simulink model "PMSM_Motor_Model_FOC_Control"  (R2021b)
settings: Solver=VariableStepAuto  StartTime=0.0  StopTime=10.0  RelTol=1e-3
undefined symbols (not defined in the file): b, DiscIntNeverNeededParam, ee_sli_rtmsupport, fsw, gcbh, idMatrix, iqMatrix, J, Ld, Lq, ModFactor, N, PM, Pmax, psim, rpmVec, Rs, Tmax, TqVec, Ts, Tsc, VdcVec
libraries: simulink x8, eeTransforms x4, eeDiscretePi x3, autolibinverter x1
settings Model: Creator=sejal  LastModifiedBy=sejal

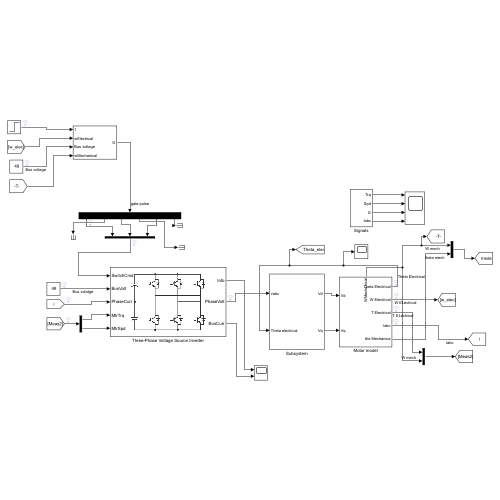
[thumbnail: Simulink's stored preview of the top-level diagram]
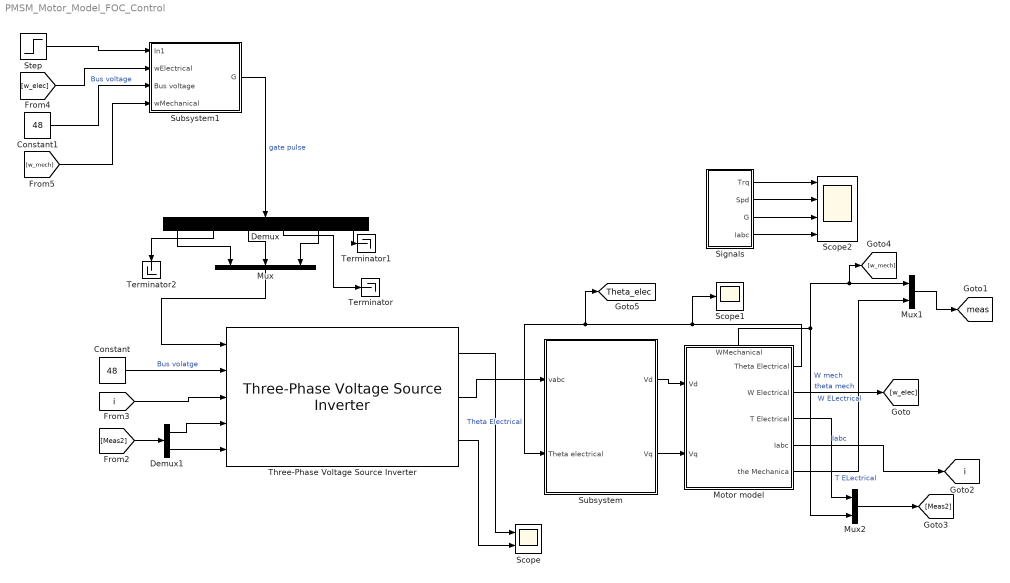
== system PMSM_Motor_Model_FOC_Control ==
  Constant : Constant  Value=48
  Constant1 : Constant  Value=48
  Demux : Demux  Outputs=6
  Demux1 : Demux  Outputs=2
  Motor model : Subsystem
      settings: PortSchema="{\"entries\":[{\"content\":{\"sides\":[{\"content\":{\"connectorIds\":[\"In1\",\"In2\"]},\"type\":\"ConnectorPlacement.EquallySpacedRectSide\",\"uuid\":\"d94b5778-ca34-457d-ba2a-6926521c1488\"},{\"content\":{\"connectorIds\":[\"Out1\",\"Out2\",\"Out3\",\"Out4\",\"Out5\"],\"side\":\"RIGHT\"},\"type\":\"ConnectorPlacement.EquallySpacedRectSide\",\"uuid\":\"5ff0fb9f-c423-410a-89d0-b078d17a40d7\"},{\"content\":{\"connectorIds\":[\"Out6\"],\"side\":\"TOP\"},\"type\":\"ConnectorPlacement.EquallySpacedRectSide\",\"uuid\":\"89b2a84c-26aa-4c46-93dc-fd6c7b13ef43\"}]},\"type\":\"ConnectorPlacement.EquallySpacedConnector\",\"uuid\":\"8745b86b-46e7-4df9-819f-71db080298ce\"}],\"packageUris\":[\"http://schema.mathworks.com/mf0/Connector/R2020b\"],\"version\":\"1.0\"}"
  Mux : Mux  Inputs=3
  Mux1 : Mux  Inputs=2
  Mux2 : Mux  Inputs=2
  Scope : Scope  NumInputPorts=2
  Scope1 : Scope
  Scope2 : Scope  NumInputPorts=4
  "Signals " : Subsystem
  Step : Step  After=500  SampleTime=0
  Subsystem : Subsystem
  Subsystem1 : Subsystem
  Terminator : Terminator
  Terminator1 : Terminator
  Terminator2 : Terminator
  Three-Phase Voltage Source Inverter : autolibinverter/Three-Phase Voltage Source Inverter  InvrtrTmpInpEnbl=off  enable_hdl=off  model_type=Switch inputs  fs=10000  w_eff_bp=[-1000 -500 0 500 1000]  n1=128  T_eff_bp=[-200 -100 0 100 200]  Temp_eff_bp=[213.15 293.15 373.15]  n2=128  ploss_table=[1 0.999 0.989 0.997 0.996;0.995 0.994 0.993 0.992 0.991;0.990 0.989 0.988 0.987 0.986;0.985 0.984 0.983 0.982 0.981;0.980 0.979 0.978 0.977 0.976]  ploss_table_3d=cat(3,0.95*[1 0.999 0.989 0.997 0.996;0.995 0.994 0.993 0.992 0.991;0.990 0.989 0.988 0.987 0.986;0.985 0.984 0.983 0.982 0.981;0.980 0.979 0.978 0.977 0.976],[1 0.999 0.989 0.997 0.996;0.995 0.994 0.993 0.992 0.991;0.990 0.989 0.988 0.987 0.986;0.985 0.984 0.983 0.982 0.981;0.980 0.979 0.978 0.977 0.976],0.92*[1 0.999 0.989 0.997 0.996;0.995 0.994 0.993 0.992 0.991;0.990 0.989 0.988 0.987 0.986;0.985 0.984 0.983 0.982 0.981;0.980 0.979 0.978 0.977 0.976])  preExtrapFlag=off  u1max=1000  u1min=-1000  u2max=200  u2min=-200  intPrec=23  RefBlkName='autolibmappedmotor/Mapped Motor'  CalLossMapData={}  CalLossWithTempMapData={}
      settings: SourceProductBaseCode=PW,DR,MT,UV,VE
  tag scope: Theta_elec=global, i=global, meas=global
  wires:
  "Signals "/2(Spd) -> Scope2/2
  "Signals "/4(Iabc) -> Scope2/4
  Motor model/6(WMechanical) -> Mux2/2, [w_mech], Mux1/1  "W mech"
  "Signals "/1(Trq) -> Scope2/1
  Three-Phase Voltage Source Inverter/2 -> Subsystem/1(vabc)
  Motor model/5(the Mechanica) -> Mux1/2  "theta mech"
  Demux/4 -> Terminator/1
  Demux/2 -> Terminator2/1
  Motor model/4(Iabc) -> [i]  "Iabc"
  Constant/1 -> Three-Phase Voltage Source Inverter/2  "Bus volatge"
  Mux2/1 -> [Meas2]
  Demux1/1 -> Three-Phase Voltage Source Inverter/4
  Demux1/2 -> Three-Phase Voltage Source Inverter/5
  [i] -> Three-Phase Voltage Source Inverter/3
  Motor model/1(Theta Electrical) -> Scope1/1, [Theta_elec], Subsystem/2(Theta electrical)  "Theta Electrical"
  Motor model/3(T Electrical) -> Mux2/1  "T ELectrical"
  Demux/1 -> Mux/1
  Demux/6 -> Terminator1/1
  Subsystem/2(Vq) -> Motor model/2(Vq)
  Three-Phase Voltage Source Inverter/3 -> Scope/2
  Three-Phase Voltage Source Inverter/1 -> Scope/1
  Subsystem/1(Vd) -> Motor model/1(Vd)
  "Signals "/3(G) -> Scope2/3
  [Meas2] -> Demux1/1
  Mux1/1 -> [meas]
  Demux/5 -> Mux/3
  Subsystem1/1(G) -> Demux/1  "gate pulse"
  Demux/3 -> Mux/2
  Mux/1 -> Three-Phase Voltage Source Inverter/1
  Motor model/2(W Electrical) -> [w_elec]  "W ELectrical"
  Step/1 -> Subsystem1/1(In1)
  [w_elec] -> Subsystem1/2(wElectrical)
  Constant1/1 -> Subsystem1/3(Bus voltage)  "Bus voltage"
  [w_mech] -> Subsystem1/4(wMechanical)

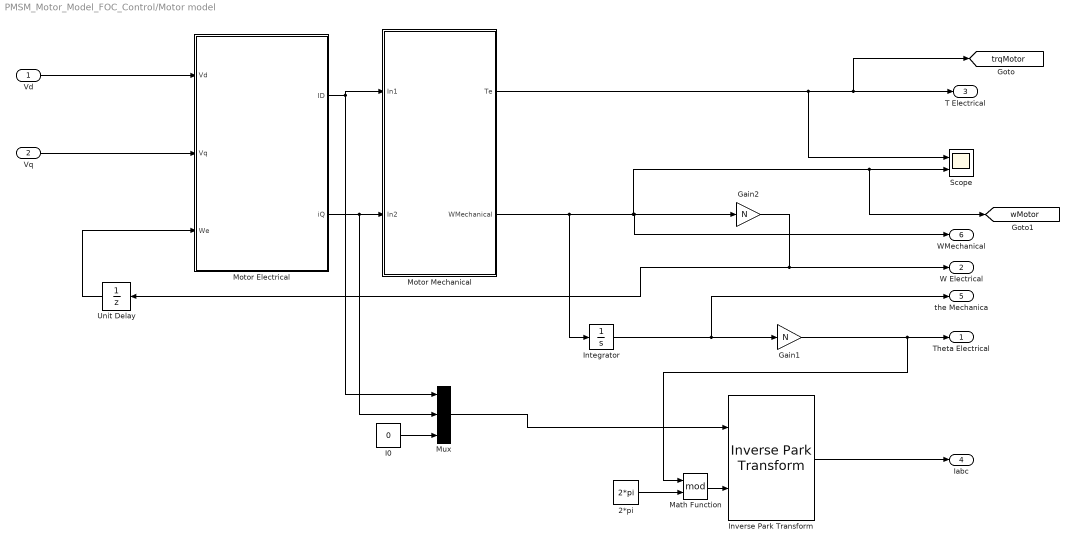
== system PMSM_Motor_Model_FOC_Control/Motor model ==
  Vd : Inport
  Vq : Inport  Port=2
  2*pi : Constant  Value=2*pi  SampleTime=Tsc
  Gain1 : Gain  Gain=N
  Gain2 : Gain  Gain=N
  I0 : Constant  Value=0
  Integrator : Integrator
  Inverse Park Transform : eeTransforms/Inverse Park Transform  AxisAlignment=Q-axis  PowerInvariant=off
  Math Function : Math  Operator=mod  SignedPower=on  SaturateOnIntegerOverflow=on
  Motor Electrical : Subsystem
  Motor Mechanical : Subsystem
  Mux : Mux  Inputs=3
  Scope : Scope  NumInputPorts=2
  Unit Delay : UnitDelay  SampleTime=-1  HasFrameUpgradeWarning=on
  Theta Electrical : Outport
  W Electrical : Outport  Port=2
  T Electrical : Outport  Port=3
  Iabc : Outport  Port=4
  the Mechanica : Outport  Port=5
  WMechanical : Outport  Port=6
  tag scope: trqMotor=global, wMotor=global
  wires:
  Motor Electrical/2(iQ) -> Mux/2, Motor Mechanical/2(In2)
  Motor Electrical/1(ID) -> Motor Mechanical/1(In1), Mux/1
  Vd/1 -> Motor Electrical/1(Vd)
  Motor Mechanical/1(Te) -> Scope/1, [trqMotor], T Electrical/1
  Vq/1 -> Motor Electrical/2(Vq)
  Integrator/1 -> the Mechanica/1, Gain1/1
  Motor Mechanical/2(WMechanical) -> WMechanical/1, Gain2/1, [wMotor], Scope/2, Integrator/1
  Mux/1 -> Inverse Park Transform/1
  I0/1 -> Mux/3
  Inverse Park Transform/1 -> Iabc/1
  Gain2/1 -> Unit Delay/1, W Electrical/1
  Unit Delay/1 -> Motor Electrical/3(We)
  2*pi/1 -> Math Function/2
  Gain1/1 -> Math Function/1, Theta Electrical/1
  Math Function/1 -> Inverse Park Transform/2

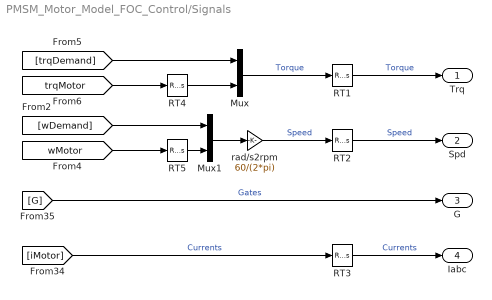
== system PMSM_Motor_Model_FOC_Control/Signals  ==
  Mux : Mux  Inputs=2
  Mux1 : Mux  Inputs=2
  RT1 : RateTransition  OutPortSampleTime=Ts
  RT2 : RateTransition  OutPortSampleTime=Ts
  RT3 : RateTransition  OutPortSampleTime=Ts
  RT4 : RateTransition  OutPortSampleTime=Tsc
  RT5 : RateTransition  OutPortSampleTime=Tsc
  rad/s2rpm : Gain  Gain=60/(2*pi)
  Trq : Outport  VectorParamsAs1DForOutWhenUnconnected=off
  Spd : Outport  Port=2  VectorParamsAs1DForOutWhenUnconnected=off
  G : Outport  Port=3  VectorParamsAs1DForOutWhenUnconnected=off
  Iabc : Outport  Port=4  VectorParamsAs1DForOutWhenUnconnected=off
  wires:
  [trqDemand] -> Mux/1
  [G] -> G/1  "Gates"
  Mux1/1 -> rad/s2rpm/1
  Mux/1 -> RT1/1  "Torque"
  [iMotor] -> RT3/1  "Currents"
  [wDemand] -> Mux1/1
  rad/s2rpm/1 -> RT2/1  "Speed"
  [trqMotor] -> RT4/1
  [wMotor] -> RT5/1
  RT1/1 -> Trq/1  "Torque"
  RT2/1 -> Spd/1  "Speed"
  RT3/1 -> Iabc/1  "Currents"
  RT4/1 -> Mux/2
  RT5/1 -> Mux1/2

== system PMSM_Motor_Model_FOC_Control/Subsystem ==
  vabc : Inport
  Theta electrical : Inport  Port=2
  2*pi : Constant  Value=2*pi  SampleTime=Tsc
  Demux1 : Demux  Outputs=3
  Math Function : Math  Operator=mod  SignedPower=on  SaturateOnIntegerOverflow=on
  Park Transform2 : eeTransforms/Park Transform  AxisAlignment=Q-axis  PowerInvariant=off
  Terminator1 : Terminator
  Trigonometric Function : Trigonometry  Commented=on
  Trigonometric Function1 : Trigonometry  Commented=on  Operator=cos
  Vd : Outport
  Vq : Outport  Port=2
  wires:
  vabc/1 -> Park Transform2/1
  Park Transform2/1 -> Demux1/1
  Demux1/3 -> Terminator1/1
  Demux1/2 -> Vq/1
  Demux1/1 -> Vd/1
  2*pi/1 -> Math Function/2
  Theta electrical/1 -> Math Function/1
  Math Function/1 -> Park Transform2/2

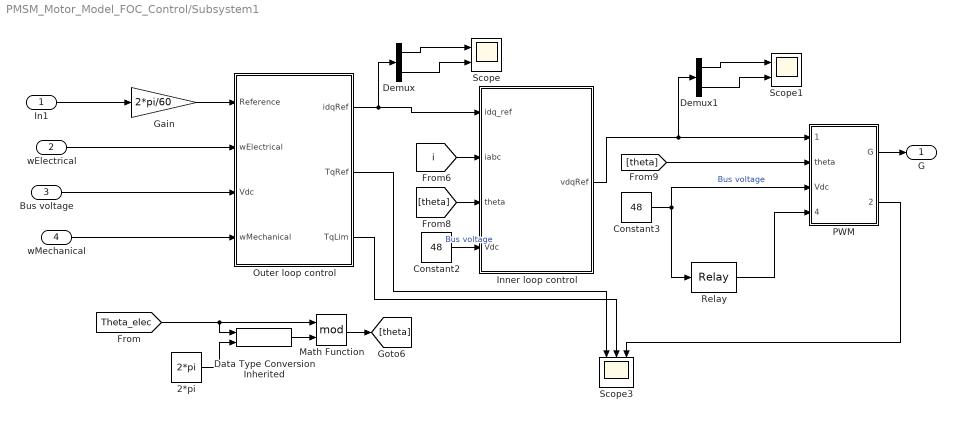
== system PMSM_Motor_Model_FOC_Control/Subsystem1 ==
  In1 : Inport
  wElectrical : Inport  Port=2
  Bus voltage : Inport  Port=3
  wMechanical : Inport  Port=4
  2*pi : Constant  Value=2*pi  OutDataTypeStr=Inherit: Inherit via back propagation  SampleTime=Tsc
  Constant2 : Constant  Value=48
  Constant3 : Constant  Value=48
  Data Type Conversion Inherited : simulink/Signal Attributes/Data Type Conversion Inherited  ConvertRealWorld=Real World Value  DoSatur=off
      settings: SourceProductBaseCode=SL
  Demux : Demux  Outputs=2
  Demux1 : Demux  Outputs=2
  Gain : Gain  Gain=2*pi/60
  Inner loop control : Subsystem  AncestorBlock=Inner_loop/Inner loop control
  Math Function : Math  Operator=mod  SignedPower=on  SaturateOnIntegerOverflow=on
  Outer loop control : Subsystem  AncestorBlock=Outer_loop/Outer loop control
  PWM : Subsystem  AncestorBlock=eePmsmFieldOrientedControl/PMSM Field-Oriented Control/PWM
  Relay : Relay  OnSwitchValue=48  OffSwitchValue=0.5*48
  Scope : Scope  NumInputPorts=2
  Scope1 : Scope  NumInputPorts=2
  Scope3 : Scope  NumInputPorts=3
  G : Outport
  wires:
  wElectrical/1 -> Outer loop control/2(wElectrical)
  [theta] -> Inner loop control/3(theta)
  Outer loop control/3(TqLim) -> Scope3/2
  Relay/1 -> PWM/4(PwmEnable)
  Data Type Conversion Inherited/1 -> Math Function/2
  In1/1 -> Gain/1
  PWM/2(ModWave) -> Scope3/3
  Gain/1 -> Outer loop control/1(Reference)
  [Theta_elec] -> Math Function/1, Data Type Conversion Inherited/1
  Outer loop control/1(idqRef) -> Demux/1, Inner loop control/1(idq_ref)
  Constant3/1 -> PWM/3(Vdc), Relay/1  "Bus voltage"
  [theta] -> PWM/2(theta)
  PWM/1(G) -> G/1
  [i] -> Inner loop control/2(iabc)
  Constant2/1 -> Inner loop control/4(Vdc)  "Bus voltage"
  2*pi/1 -> Data Type Conversion Inherited/2
  Outer loop control/2(TqRef) -> Scope3/1
  Math Function/1 -> [theta]
  wMechanical/1 -> Outer loop control/4(wMechanical)
  Bus voltage/1 -> Outer loop control/3(Vdc)
  Demux/1 -> Scope/1
  Demux/2 -> Scope/2
  Demux1/1 -> Scope1/1
  Inner loop control/1(vdqRef) -> Demux1/1, PWM/1(vdqRef)
  Demux1/2 -> Scope1/2

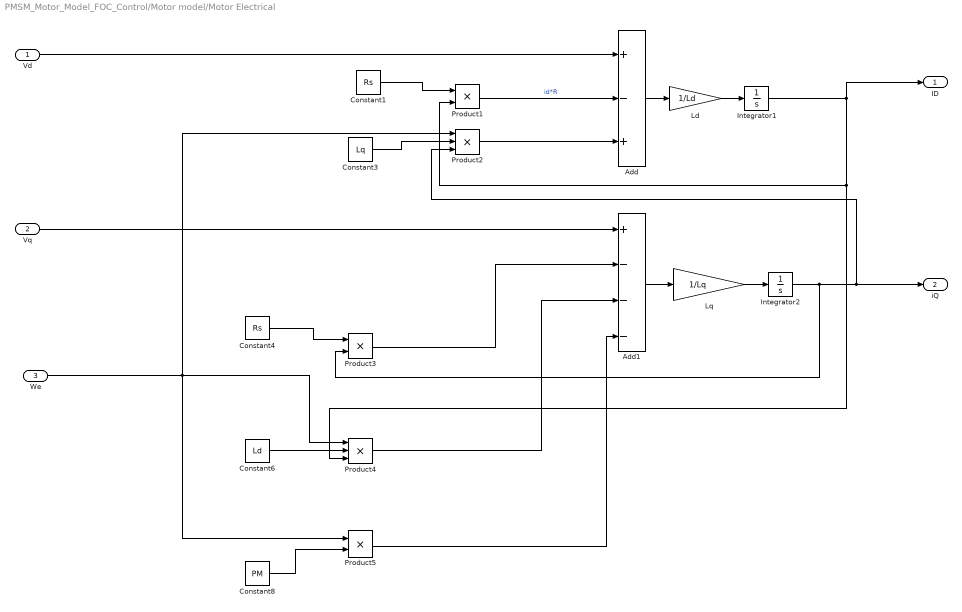
== system PMSM_Motor_Model_FOC_Control/Motor model/Motor Electrical ==
  Vd : Inport
  Vq : Inport  Port=2
  We : Inport  Port=3
  Add : Sum  Inputs=+-+
  Add1 : Sum  Inputs=+---
  Constant1 : Constant  Value=Rs
  Constant3 : Constant  Value=Lq
  Constant4 : Constant  Value=Rs
  Constant6 : Constant  Value=Ld
  Constant8 : Constant  Value=PM
  Integrator1 : Integrator
  Integrator2 : Integrator
  Ld : Gain  Gain=1/Ld
  Lq : Gain  Gain=1/Lq
  Product1 : Product
  Product2 : Product  Inputs=3
  Product3 : Product
  Product4 : Product  Inputs=3
  Product5 : Product
  ID : Outport
  iQ : Outport  Port=2
  wires:
  Constant3/1 -> Product2/2
  Add/1 -> Ld/1
  Product5/1 -> Add1/4
  Integrator2/1 -> Product2/3, iQ/1, Product3/2
  Constant8/1 -> Product5/2
  Constant1/1 -> Product1/1
  Product1/1 -> Add/2  "id*R"
  Product2/1 -> Add/3
  Add1/1 -> Lq/1
  We/1 -> Product5/1, Product2/1, Product4/1
  Constant4/1 -> Product3/1
  Lq/1 -> Integrator2/1
  Product3/1 -> Add1/2
  Constant6/1 -> Product4/2
  Product4/1 -> Add1/3
  Vd/1 -> Add/1
  Vq/1 -> Add1/1
  Integrator1/1 -> Product1/2, Product4/3, ID/1
  Ld/1 -> Integrator1/1

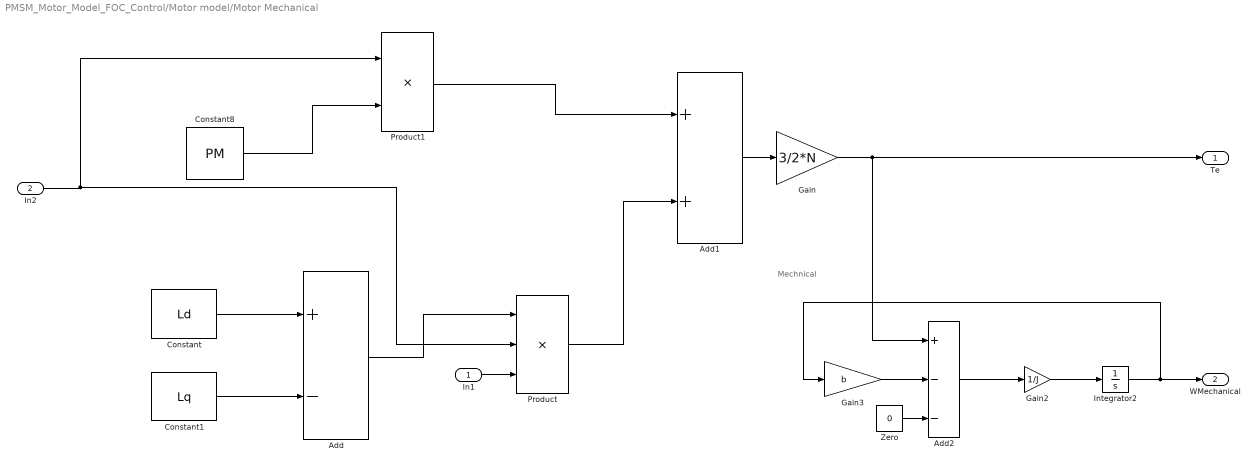
== system PMSM_Motor_Model_FOC_Control/Motor model/Motor Mechanical ==
  note: Mechnical
  In1 : Inport
  In2 : Inport  Port=2
  Add : Sum  Inputs=+-
  Add1 : Sum
  Add2 : Sum  Inputs=+--
  Constant : Constant  Value=Ld
  Constant1 : Constant  Value=Lq
  Constant8 : Constant  Value=PM
  Gain : Gain  Gain=3/2*N
  Gain2 : Gain  Gain=1/J
  Gain3 : Gain  Gain=b
  Integrator2 : Integrator
  Product : Product  Inputs=3
  Product1 : Product
  Zero : Constant  Value=0  OutDataTypeStr=Inherit: Inherit via back propagation
  Te : Outport
  WMechanical : Outport  Port=2
  wires:
  Add1/1 -> Gain/1
  Constant8/1 -> Product1/2
  Constant/1 -> Add/1
  Add/1 -> Product/1
  Constant1/1 -> Add/2
  Product1/1 -> Add1/1
  Product/1 -> Add1/2
  In2/1 -> Product/2, Product1/1
  In1/1 -> Product/3
  Gain/1 -> Te/1, Add2/1
  Zero/1 -> Add2/3
  Gain3/1 -> Add2/2
  Integrator2/1 -> WMechanical/1, Gain3/1
  Add2/1 -> Gain2/1
  Gain2/1 -> Integrator2/1

== system PMSM_Motor_Model_FOC_Control/Subsystem1/Inner loop control ==
  idq_ref : Inport
  iabc : Inport  Port=2
  theta : Inport  Port=3
  Vdc : Inport  Port=4
  Constant : Constant  Value=0  SampleTime=-1
  Gain : Gain  Gain=1/sqrt(3)
  PMSM Current Controller : Subsystem  AncestorBlock=eePmsmCurrentController/PMSM Current Controller  LoadFcn=ee_sli_rtmsupport( 'loadfcn', gcbh );  mask(PMSM Current Controller){Kp_id=0.1, Ki_id=10, Kaw_id=1000, Kp_iq=0.1, Ki_iq=10, Kaw_iq=1000, Ts=-1, Tsd=0.001, AxisPrio=Q-axis, ActZC=off, ActFF=on}
      mask prompts: Kp_id "physmod:ee:library:comments:control:eePmsmCurrentController:DaxisCurrentProportionalGain_MP"; Ki_id "physmod:ee:library:comments:control:eePmsmCurrentController:DaxisCurrentIntegralGain_MP"; Kaw_id "physmod:ee:library:comments:control:eePmsmCurrentController:DaxisCurrentAntiwindupGain_MP"; Kp_iq "physmod:ee:library:comments:control:eePmsmCurrentController:QaxisCurrentProportionalGain_MP"; Ki_iq "physmod:ee:library:comments:control:eePmsmCurrentController:QaxisCurrentIntegralGain_MP"; Kaw_iq "physmod:ee:library:comments:control:eePmsmCurrentController:QaxisCurrentAntiwindupGain_MP"; Ts "physmod:ee:library:comments:control:eePmsmCurrentController:SampleTime1ForInherited_MP"; Tsd "physmod:ee:library:comments:control:eePmsmCurrentController:DiscretizationSampleTime_MP"; AxisPrio "physmod:ee:library:comments:control:eePmsmCurrentController:AxisPrioritization_MP"; ActZC "physmod:ee:library:comments:control:eePmsmCurrentController:EnableZeroCancellation_MP"; ActFF "physmod:ee:library:comments:control:eePmsmCurrentController:EnablePrecontrolVoltage_MP"
      mask help: physmod:ee:library:comments:control:eePmsmCurrentController:PMSMCurrentController_MD
      mask init:
      | [Tsd, numZC_id, denZC_id, numZC_iq, denZC_iq] = ee.mask.initializePmsmCurrentController(ActZC,Ts,Tsd,Kp_id,Ki_id,Kp_iq,Ki_iq);
      settings: CopyFcn=ee_sli_rtmsupport( 'copyfcn', gcbh );  DeleteFcn=ee_sli_rtmsupport( 'deletefcn', gcbh );  ModelCloseFcn=ee_sli_rtmsupport( 'modelclosefcn', gcbh );  PostSaveFcn=ee_sli_rtmsupport( 'postsavefcn', gcbh );  PreCopyFcn=ee_sli_rtmsupport( 'precopyfcn', gcbh );  OpenFcn=ee_sli_rtmsupport( 'openfcn', gcbh );  CloseFcn=ee_sli_rtmsupport( 'closefcn', gcbh );  PreDeleteFcn=ee_sli_rtmsupport( 'predeletefcn', gcbh );
      mask Help: web(nesl_help(gcbh))
      mask Callback Ts: ee.mask.callbackZeroCancellation(gcb);
      mask TypeOptions AxisPrio: d-q Voltage Limiter/AxisPrio
      mask Callback ActZC: ee.mask.callbackZeroCancellation(gcb);
      mask DialogControl Container1 Prompt: physmod:ee:library:comments:control:eePmsmCurrentController:tab_ControlParameters
      mask DialogControl Kp_id Prompt: D-axis current proportional gain
      mask DialogControl Ki_id Prompt: D-axis current integral gain
      mask DialogControl Kaw_id Prompt: D-axis current anti-windup gain
      mask DialogControl Kp_iq Prompt: Q-axis current proportional gain
      mask DialogControl Ki_iq Prompt: Q-axis current integral gain
      mask DialogControl Kaw_iq Prompt: Q-axis current anti-windup gain
      mask DialogControl Ts Prompt: Sample time (-1 for inherited)
      mask DialogControl Tsd Prompt: Discretization sample time
      mask DialogControl AxisPrio Prompt: Axis prioritization
      mask DialogControl ActZC Prompt: Enable zero cancellation
      mask DialogControl ActFF Prompt: Enable pre-control voltage
  Park Transform : eeTransforms/Park Transform  AxisAlignment=Q-axis  PowerInvariant=off
  vdqRef : Outport  VectorParamsAs1DForOutWhenUnconnected=off
  wires:
  idq_ref/1 -> PMSM Current Controller/1(idqRef)
  iabc/1 -> Park Transform/1
  Vdc/1 -> Gain/1
  PMSM Current Controller/1(vdqRef) -> vdqRef/1
  theta/1 -> Park Transform/2
  Park Transform/1 -> PMSM Current Controller/2(idq)
  Constant/1 -> PMSM Current Controller/4(Reset)
  Gain/1 -> PMSM Current Controller/3(VphMax)

== system PMSM_Motor_Model_FOC_Control/Subsystem1/Outer loop control ==
  Reference : Inport
  wElectrical : Inport  Port=2
  Vdc : Inport  Port=3
  wMechanical : Inport  Port=4  SampleTime=Ts
  Discrete PI Controller : eeDiscretePi/Discrete PI Controller  Kp=60  Ki=300*2  Kaw=1000  x0=0  Ts=Ts
      settings: SourceProductBaseCode=PS
  PMSM Current Reference Generator : Subsystem  AncestorBlock=eePmsmCurrentReferenceGen/PMSM Current Reference Generator  LoadFcn=ee_sli_rtmsupport( 'loadfcn', gcbh );  mask(PMSM Current Reference Generator){Vnom=48, Pmax=Pmax, Tmax=Tmax, Ts=Tsc, RefType=Zero d-axis control, rpmVec=rpmVec, TqVec=TqVec, VdcVec=VdcVec, PWMMode=SVM: space vector modulation, ModFactor=ModFactor, idMatrix=idMatrix, iqMatrix=iqMatrix, p=N, psim=psim, Ld=Ld, Lq=Lq, Rs=Rs, RefExpEnable=0}
      mask prompts: Vnom "physmod:ee:library:comments:control:eePmsmCurrentReferenceGen:NominalDclinkVoltageV_MP"; Pmax "physmod:ee:library:comments:control:eePmsmCurrentReferenceGen:MaximumPowerW_MP"; Tmax "physmod:ee:library:comments:control:eePmsmCurrentReferenceGen:MaximumTorqueNm_MP"; Ts "physmod:ee:library:comments:control:eePmsmCurrentReferenceGen:SampleTime1ForInherited_MP"; RefType "physmod:ee:library:comments:control:eePmsmCurrentReferenceGen:CurrentReferences_MP"; rpmVec "physmod:ee:library:comments:control:eePmsmCurrentReferenceGen:MechanicalSpeedVectorWMechanicalrpm_MP"; TqVec "physmod:ee:library:comments:control:eePmsmCurrentReferenceGen:TorqueReferenceVectorTqRefNm_MP"; VdcVec "physmod:ee:library:comments:control:eePmsmCurrentReferenceGen:DClinkVoltageVectorVdcV_MP"; PWMMode "physmod:ee:library:comments:control:eePmsmCurrentReferenceGen:PWMMethod_MP"; ModFactor "physmod:ee:library:comments:control:eePmsmCurrentReferenceGen:ModulationFactor_MP"; idMatrix "physmod:ee:library:comments:control:eePmsmCurrentReferenceGen:DaxisCurrentReferenceMatrixIdwMechanicalTqRefVdcA_MP"; iqMatrix "physmod:ee:library:comments:control:eePmsmCurrentReferenceGen:QaxisCurrentReferenceMatrixIqwMechanicalTqRefVdcA_MP"; p "physmod:ee:library:comments:control:eePmsmCurrentReferenceGen:NumberOfRotorPolePairs_MP"; psim "physmod:ee:library:comments:control:eePmsmCurrentReferenceGen:PermanentMagnetFluxLinkageWb_MP"; Ld "physmod:ee:library:comments:control:eePmsmCurrentReferenceGen:DaxisInductanceH_MP"; Lq "physmod:ee:library:comments:control:eePmsmCurrentReferenceGen:QaxisInductanceH_MP"; Rs "physmod:ee:library:comments:control:eePmsmCurrentReferenceGen:StatorResistanceOhm_MP"; RefExpEnable "physmod:ee:library:comments:control:eePmsmCurrentReferenceGen:ExportCurrentReferences_MP"
      mask help: physmod:ee:library:comments:control:eePmsmCurrentReferenceGen:PMSMCurrentReferenceGenerator_MD
      mask init:
      | if Vnom <= 0            
      |     error(message('physmod:simscape:compiler:patterns:checks:GreaterThanZero',getString(message('physmod:ee:library:comments:control:eePmsmCurrentReferenceGen:NominalDclinkVoltageV_MP'))));            
      | end
      | if Pmax <= 0            
      |     error(message('physmod:simscape:compiler:patterns:checks:GreaterThanZero',getString(message('physmod:ee:library:comments:control:eePmsmCurrentReferenceGen:MaximumPowerW_MP'))));            
      | end
      | if Tmax <= 0            
      |     error(message('physmod:simscape:compiler:patterns:checks:GreaterThanZero',getString(message('physmod:ee:library:comments:control:eePmsmCurrentReferenceGen:MaximumTorqueNm_MP'))));            
      | end
      | switch RefType
      |     case 'Zero d-axis control'
      |         EnableZDAC = 1;
      |         rpmVec = [0, 3000];
      |         TqVec  = [-100, 0, 100];
      |         VdcVec = [300, 350];
      |         idMatrix = zeros(2,3,2);
      |         iqMatrix = zeros(2,3,2);
      |     case 'Lookup-table based'
      |         EnableZDAC = 0;
      |         if length(rpmVec) < 2            
      |             error(message('physmod:simscape:compiler:patterns:checks:LengthGreaterThanOrEqual',getString(message('physmod:ee:library:comments:control:eePmsmCurrentReferenceGen:MechanicalSpeedVectorWMechanicalrpm_MP')), '2'));            
      |         end
      |         if ~all(diff(rpmVec) > 0)            
      |             error(message('physmod:simscape:compiler:patterns:checks:StrictlyAscendingVec',getString(message('physmod:ee:library:comments:control:eePmsmCurrentReferenceGen:MechanicalSpeedVectorWMechanicalrpm_MP'))));            
      |         end
      |         if length(TqVec) < 2            
      |             error(message('physmod:simscape:compiler:patterns:checks:LengthGreaterThanOrEqual',getString(message('physmod:ee:library:comments:control:eePmsmCurrentReferenceGen:TorqueReferenceVectorTqRefNm_MP')), '2'));            
      |         end
      |         if ~all(diff(TqVec) > 0)            
      |             error(message('physmod:simscape:compiler:patterns:checks:StrictlyAscendingVec',getString(message('physmod:ee:library:comments:control:eePmsmCurrentReferenceGen:TorqueReferenceVectorTqRefNm_MP'))));            
      |         end
      |         if length(VdcVec) < 2            
      |             error(message('physmod:simscape:compiler:patterns:checks:LengthGreaterThanOrEqual',getString(message('physmod:ee:library:comments:control:eePmsmCurrentReferenceGen:DClinkVoltageVectorVdcV_MP')), '2'));            
      |         end
      |         if ~all(diff(VdcVec) > 0)            
      |             error(message('physmod:simscape:compiler:patterns:checks:StrictlyAscendingVec',getString(message('physmod:ee:library:comments:control:eePmsmCurrentReferenceGen:DClinkVoltageVectorVdcV_MP'))));            
      |         end
      |         if ~all(size(idMatrix) == [length(rpmVec), length(TqVec), length(VdcVec)])            
      |             error(message('physmod:simscape:compiler:patterns:checks:Size3DEqual',getString(message('physmod:ee:library:comments:control:eePmsmCurrentReferenceGen:DaxisCurrentReferenceMatrixIdwMechanicalTqRefVdcA_MP')), getString(message('physmod:ee:library:comments:control:eePmsmCurrentReferenceGen:MechanicalSpeedVectorWMechanicalrpm_MP')), getString(message('physmod:ee:library:comments:control:eePmsmCurrentReferenceGen:TorqueReferenceVectorTqRefNm_MP')), getString(message('physmod:ee:library:comments:control:eePmsmCurrentReferenceGen:DClinkVoltageVectorVdcV_MP'))));            
      |         end
      |         if ~all(size(iqMatrix) == [length(rpmVec), length(TqVec), length(VdcVec)])            
      |             error(message('physmod:simscape:compiler:patterns:checks:Size3DEqual',getString(message('physmod:ee:library:comments:control:eePmsmCurrentReferenceGen:QaxisCurrentReferenceMatrixIqwMechanicalTqRefVdcA_MP')), getString(message('physmod:ee:library:comments:control:eePmsmCurrentReferenceGen:MechanicalSpeedVectorWMechanicalrpm_MP')), getString(message('physmod:ee:library:comments:control:eePmsmCurrentReferenceGen:TorqueReferenceVectorTqRefNm_MP')), getString(message('physmod:ee:library:comments:control:eePmsmCurrentReferenceGen:DClinkVoltageVectorVdcV_MP'))));            
      |         end
      |     case 'Automatically generated lookup-table'
      |         EnableZDAC = 0;
      |         if Rs <= 0            
      |             error(message('physmod:simscape:compiler:patterns:checks:GreaterThanZero',getString(message('physmod:ee:library:comments:control:eePmsmCurrentReferenceGen:StatorResistanceOhm_MP'))));            
      |         end
      |         if Ld <= 0            
      |             error(message('physmod:simscape:compiler:patterns:checks:GreaterThanZero',getString(message('physmod:ee:library:comments:control:eePmsmCurrentReferenceGen:DaxisInductanceH_MP'))));            
      |         end
      |         if Lq <= 0            
      |             error(message('physmod:simscape:compiler:patterns:checks:GreaterThanZero',getString(message('physmod:ee:library:comments:control:eePmsmCurrentReferenceGen:QaxisInductanceH_MP'))));            
      |         end
      |         
      |         if ModFactor <= 0            
      |             error(message('physmod:simscape:compiler:patterns:checks:GreaterThanZero',getString(message('physmod:ee:library:comments:control:eePmsmCurrentReferenceGen:ModulationFactor_MP'))));            
      |         end
      |         
      |         if ModFactor > 1            
      |             error(message('physmod:simscape:compiler:patterns:checks:LessThanOrEqual',getString(message('physmod:ee:library:comments:control:eePmsmCurrentReferenceGen:ModulationFactor_MP')),'1'));            
      |         end
      |         
      |         % Check if machine parameters were changed
      |         if exist('pmsm_data', 'var')
      |             dataUpdate = (pmsm_data.Ld   ~= Ld)   ||...
      |                          (pmsm_data.Lq   ~= Lq)   ||...
      |                          (pmsm_data.psim ~= psim) ||...
      |                          (pmsm_data.p    ~= p)    ||...
      |                          (pmsm_data.Rs   ~= Rs)   ||...
      |                          (pmsm_data.Pmax ~= Pmax) ||...
      |                          (pmsm_data.Tmax ~= Tmax) ||...
      |                          (pmsm_data.PWMMode ~= PWMMode) ||...
      |                          (pmsm_data.ModFactor ~= ModFactor);
      |         end
      |         % Check if grid points were changed
      |         if exist('grid_points', 'var')
      |             VecUpdate = max(abs(grid_points.RPM_VECT - rpmVec))~=0 ||...
      |                         max(abs(grid_points.TQ_VECT  - TqVec)) ~=0 ||...
      |                         max(abs(grid_points.VDC_VECT - VdcVec))~=0;
      |         end
      |         % Compute current references only IF current references do not exist OR 
      |         % machine parameters were changed OR grid points were changed
      |         if ~exist('pmsm_ref', 'var') || dataUpdate || VecUpdate
      |             grid_points.RPM_VECT = rpmVec;
      |             grid_points.TQ_VECT  = TqVec;
      |             grid_points.VDC_VECT = VdcVec;
      |             pmsm_data.Ld    = Ld; 
      |             pmsm_data.Lq    = Lq; 
      |             pmsm_data.psim  = psim;   
      |             pmsm_data.p     = p;         
      |             pmsm_data.Rs    = Rs;   
      |             pmsm_data.Pmax  = Pmax;      
      |             pmsm_data.Tbase = Tmax;    
      |             pmsm_data.PWMMode   = PWMMode;      
      |             pmsm_data.ModFactor = ModFactor;
      |             pmsm_ref = ee.control.pmsm.getCurrentReferencesPmsm ( pmsm_data, grid_points );
      |             idMatrix = pmsm_ref.idMatrix;
      |             iqMatrix = pmsm_ref.iqMatrix;
      |         end
      |         % Export current references to base workspace
      |         if RefExpEnable==1
      |             assignin('base', 'pmsm_ref', pmsm_ref)
      |             set_param(gcb,'RefExpEnable','0');
      |         end
      | end
      settings: CopyFcn=ee_sli_rtmsupport( 'copyfcn', gcbh );  DeleteFcn=ee_sli_rtmsupport( 'deletefcn', gcbh );  ModelCloseFcn=ee_sli_rtmsupport( 'modelclosefcn', gcbh );  PostSaveFcn=ee_sli_rtmsupport( 'postsavefcn', gcbh );  PreCopyFcn=ee_sli_rtmsupport( 'precopyfcn', gcbh );  OpenFcn=ee_sli_rtmsupport( 'openfcn', gcbh );  CloseFcn=ee_sli_rtmsupport( 'closefcn', gcbh );  PreDeleteFcn=ee_sli_rtmsupport( 'predeletefcn', gcbh );
      mask Help: web(nesl_help(gcbh))
      mask TypeOptions RefType: physmod:ee:library:comments:control:eePmsmCurrentReferenceGen:ZeroD0x2DAxisControl_PV | physmod:ee:library:comments:control:eePmsmCurrentReferenceGen:Lookup0x2DTableBased_PV | physmod:ee:library:comments:control:eePmsmCurrentReferenceGen:AutomaticallyGeneratedLookup0x2DTable_PV
      mask Callback RefType:
      | % Callback function to set the parameters visibility
      | ee.mask.callbackPopupRefGenPmsm(gcb);
      mask TypeOptions PWMMode: physmod:ee:library:comments:control:eePmsmCurrentReferenceGen:SPWMSinusoidalPWM_PV | physmod:ee:library:comments:control:eePmsmCurrentReferenceGen:SVMSpaceVectorModulation_PV
      mask DialogControl Container2 Prompt: physmod:ee:library:comments:control:eePmsmCurrentReferenceGen:tab_GeneralParameters
      mask DialogControl Vnom Prompt: Nominal dc-link voltage (V)
      mask DialogControl Pmax Prompt: Maximum power (W)
      mask DialogControl Tmax Prompt: Maximum torque (N*m)
      mask DialogControl Ts Prompt: Sample time (-1 for inherited)
      mask DialogControl Container3 Prompt: physmod:ee:library:comments:control:eePmsmCurrentReferenceGen:tab_ReferenceGenStrategy
      mask DialogControl RefType Prompt: Current references
      mask DialogControl rpmVec Prompt: Mechanical speed vector, wMechanical (rpm)
      mask DialogControl TqVec Prompt: Torque reference vector, TqRef (N*m)
      mask DialogControl VdcVec Prompt: DC-link voltage vector, Vdc (V)
      mask DialogControl PWMMode Prompt: PWM method
      mask DialogControl ModFactor Prompt: Modulation factor
      mask DialogControl idMatrix Prompt: D-axis current reference matrix, id(wMechanical,TqRef,Vdc), (A)
      mask DialogControl iqMatrix Prompt: Q-axis current reference matrix, iq(wMechanical,TqRef,Vdc), (A)
      mask DialogControl p Prompt: Number of rotor pole pairs
      mask DialogControl psim Prompt: Permanent magnet flux linkage (Wb)
      mask DialogControl Ld Prompt: D-axis inductance (H)
      mask DialogControl Lq Prompt: Q-axis inductance (H)
      mask DialogControl Rs Prompt: Stator resistance (Ohm)
      mask DialogControl RefExp Prompt: physmod:ee:library:comments:control:eePmsmCurrentReferenceGen:ExportCurrentReferencesToWorkspace_B
      mask DialogControl RefExp Callback:
      | % Enable export of current references
      | set_param(gcb,'RefExpEnable','1');
      mask DialogControl RefExpEnable Prompt: Export current references
  Sum : Sum  Inputs=|+-
  Zero : Constant  Value=0  OutDataTypeStr=Inherit: Inherit via back propagation
  elec->mech : Gain  Gain=1/N
  idqRef : Outport  VectorParamsAs1DForOutWhenUnconnected=off
  TqRef : Outport  Port=2  VectorParamsAs1DForOutWhenUnconnected=off
  TqLim : Outport  Port=3  VectorParamsAs1DForOutWhenUnconnected=off
  wires:
  wMechanical/1 -> Sum/2
  Sum/1 -> Discrete PI Controller/1
  Zero/1 -> Discrete PI Controller/3, Discrete PI Controller/2
  Discrete PI Controller/1 -> PMSM Current Reference Generator/1(TqRef)  "Torque reference"
  Reference/1 -> Sum/1
  wElectrical/1 -> elec->mech/1
  Vdc/1 -> PMSM Current Reference Generator/3(Vdc)
  PMSM Current Reference Generator/1(idqRef) -> idqRef/1
  PMSM Current Reference Generator/2(TqRefSat) -> TqRef/1
  PMSM Current Reference Generator/3(TqLim) -> TqLim/1
  elec->mech/1 -> PMSM Current Reference Generator/2(wMechanical)

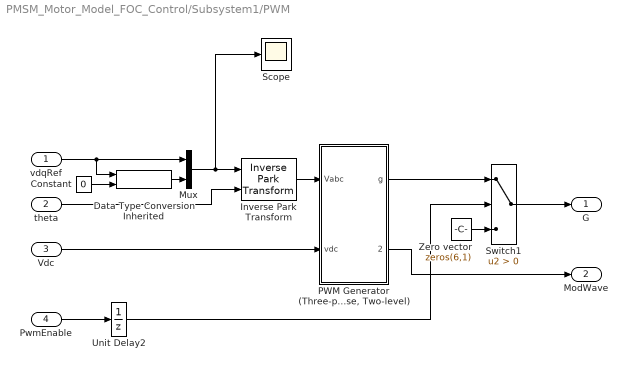
== system PMSM_Motor_Model_FOC_Control/Subsystem1/PWM ==
  vdqRef : Inport
  theta : Inport  Port=2
  Vdc : Inport  Port=3
  PwmEnable : Inport  Port=4
  Constant : Constant  Value=0  SampleTime=Tsc
  Data Type Conversion Inherited : simulink/Signal Attributes/Data Type Conversion Inherited  ConvertRealWorld=Real World Value  DoSatur=off
      settings: SourceProductBaseCode=SL
  Inverse Park Transform : eeTransforms/Inverse Park Transform  AxisAlignment=Q-axis  PowerInvariant=off
  Mux : Mux  Inputs=2
  "PWM Generator (Three-phase, Two-level)" : Subsystem  AncestorBlock=|  LoadFcn=ee_sli_rtmsupport( 'loadfcn', gcbh );  mask(PWM Generator (three-phase, two-level)){PWMMode=Continuous PWM (CPWM), CPWMMode=SPWM: sinusoidal PWM, DPWMMode=60 DPWM: 60 degree discontinuous PWM, SamplingMode=Natural, fsw=fsw, Ts=Ts}
      | eePwmGeneratorTwoLevel/PWM Generator
      | (Three-phase, Two-level)
      mask prompts: PWMMode "physmod:ee:library:comments:control:eePwmGeneratorTwoLevel:PWMMode_MP"; CPWMMode "physmod:ee:library:comments:control:eePwmGeneratorTwoLevel:ContinuousPWM_MP"; DPWMMode "physmod:ee:library:comments:control:eePwmGeneratorTwoLevel:DiscontinuousPWM_MP"; SamplingMode "physmod:ee:library:comments:control:eePwmGeneratorTwoLevel:SamplingMode_MP"; fsw "physmod:ee:library:comments:control:eePwmGeneratorTwoLevel:SwitchingFrequencyHz_MP"; Ts "physmod:ee:library:comments:control:eePwmGeneratorTwoLevel:SampleTimes_MP"
      mask help: physmod:ee:library:comments:control:eePwmGeneratorTwoLevel:PWMGeneratorthreephaseTwolevel_MD
      mask init:
      | Tsw = 1/fsw;
      | 
      | if fsw <= 0
      |     error(message('physmod:simscape:compiler:patterns:checks:GreaterThanZero',getString(message('physmod:ee:library:comments:control:eePwmGeneratorTwoLevel:SwitchingFrequencyHz_MP'))));
      | end
      | 
      | if Ts <= 0
      |     error(message('physmod:simscape:compiler:patterns:checks:GreaterThanZero',getString(message('physmod:ee:library:comments:control:eePwmGeneratorTwoLevel:SampleTimes_MP'))));
      | end
      | 
      | if Ts > 1/(10*fsw)
      |     error(message('physmod:simscape:compiler:patterns:checks:LessThanOrEqual',getString(message('physmod:ee:library:comments:control:eePwmGeneratorTwoLevel:SampleTimes_MP')),getString(message('physmod:ee:library:comments:control:eePwmGeneratorTwoLevel:inverseOf10TimesSwitchingFrequency_MP'))));
      | end
      | 
      | switch SamplingMode
      |     case 'Natural'
      |         RateTransitionOnInput = -1;
      |         GateGeneratorX0 = 0;
      |     case 'Asymmetric'
      |         RateTransitionOnInput = 0.5*Tsw;
      |         GateGeneratorX0 = 0.5/fsw;
      |     case 'Symmetric'
      |         RateTransitionOnInput = Tsw;
      |         GateGeneratorX0 = 0;
      | end
      | 
      | 
      | switch PWMMode
      |     case 'Continuous PWM (CPWM)'
      |         switch CPWMMode
      |             case 'SPWM: sinusoidal PWM'
      |                 PWM = 1;
      |             case 'SVM: space vector modulation'
      |                 PWM = 2;
      |         end
      |     case 'Discontinuous PWM (DPWM)'
      |         switch DPWMMode
      |             case '60 DPWM: 60 degree discontinuous PWM'
      |                 PWM = 3;
      |             case '60 DPWM (+30 degree shift): +30 degree shift from 60 DPWM'
      |                 PWM = 4;
      |             case '60 DPWM (-30 degree shift): -30 degree shift from 60 DPWM'
      |                 PWM = 5;
      |             case '30 DPWM: 30 degree discontinuous PWM'
      |                 PWM = 6;
      |             case '120 DPWM: positive dc component'
      |                 PWM = 7;
      |             case '120 DPWM: negative dc component'
      |                 PWM = 8;
      |         end
      | end
      settings: CopyFcn=ee_sli_rtmsupport( 'copyfcn', gcbh );  DeleteFcn=ee_sli_rtmsupport( 'deletefcn', gcbh );  ModelCloseFcn=ee_sli_rtmsupport( 'modelclosefcn', gcbh );  PreSaveFcn=%pe_sli_rtmsupport( 'presavefcn', gcbh );  PostSaveFcn=ee_sli_rtmsupport( 'postsavefcn', gcbh );  PreCopyFcn=ee_sli_rtmsupport( 'precopyfcn', gcbh );  OpenFcn=ee_sli_rtmsupport( 'openfcn', gcbh );  CloseFcn=ee_sli_rtmsupport( 'closefcn', gcbh );  PreDeleteFcn=ee_sli_rtmsupport( 'predeletefcn', gcbh );
      mask Help: web(nesl_help(gcbh))
      mask TypeOptions PWMMode: physmod:ee:library:comments:control:eePwmGeneratorTwoLevel:ContinuousPWMCPWM_PV | physmod:ee:library:comments:control:eePwmGeneratorTwoLevel:DiscontinuousPWMDPWM_PV
      mask Callback PWMMode:
      | switch get_param(gcb,'PWMMode')
      |     case 'Continuous PWM (CPWM)'
      |         set_param(gcb,'MaskVisibilities',{'on';'on';'off';'on';'on';'on'})
      |     case 'Discontinuous PWM (DPWM)'
      |         set_param(gcb,'MaskVisibilities',{'on';'off';'on';'on';'on';'on'})
      | end
      mask TypeOptions CPWMMode: physmod:ee:library:comments:control:eePwmGeneratorTwoLevel:SPWMSinusoidalPWM_PV | physmod:ee:library:comments:control:eePwmGeneratorTwoLevel:SVMSpaceVectorModulation_PV
      mask TypeOptions DPWMMode: physmod:ee:library:comments:control:eePwmGeneratorTwoLevel:x60DPWM60DegreeDiscontinuousPWM_PV | physmod:ee:library:comments:control:eePwmGeneratorTwoLevel:x60DPWM30DegreeShift30DegreeShiftFrom60DPWM_PV | physmod:ee:library:comments:control:eePwmGeneratorTwoLevel:x60DPWM0x2D30DegreeShift0x2D30DegreeShiftFrom60DPWM_PV | physmod:ee:library:comments:control:eePwmGeneratorTwoLevel:x30DPWM30DegreeDiscontinuousPWM_PV | physmod:ee:library:comments:control:eePwmGeneratorTwoLevel:x120DPWMPositiveDcComponent_PV | physmod:ee:library:comments:control:eePwmGeneratorTwoLevel:x120DPWMNegativeDcComponent_PV
      mask TypeOptions SamplingMode: physmod:ee:library:comments:control:eePwmGeneratorTwoLevel:Natural_PV | physmod:ee:library:comments:control:eePwmGeneratorTwoLevel:Asymmetric_PV | physmod:ee:library:comments:control:eePwmGeneratorTwoLevel:Symmetric_PV
      mask DialogControl ParameterGroupVar Prompt: physmod:ee:library:comments:control:eePwmGeneratorTwoLevel:tab_Parameters
      mask DialogControl PWMMode Prompt: PWM mode
      mask DialogControl CPWMMode Prompt: Continuous PWM
      mask DialogControl DPWMMode Prompt: Discontinuous PWM
      mask DialogControl SamplingMode Prompt: Sampling mode
      mask DialogControl fsw Prompt: Switching frequency (Hz)
      mask DialogControl Ts Prompt: Sample time (s)
  Scope : Scope
  Switch1 : Switch  Criteria=u2 > Threshold
  Unit Delay2 : UnitDelay  SampleTime=Tsc  HasFrameUpgradeWarning=on
  Zero vector : Constant  Value=zeros(6,1)  SampleTime=Ts
  G : Outport  VectorParamsAs1DForOutWhenUnconnected=off
  ModWave : Outport  Port=2  SampleTime=Tsc  VectorParamsAs1DForOutWhenUnconnected=off
  wires:
  Constant/1 -> Data Type Conversion Inherited/2
  Data Type Conversion Inherited/1 -> Mux/2
  Unit Delay2/1 -> Switch1/2
  Vdc/1 -> "PWM Generator (Three-phase, Two-level)"/2(vdc)
  Inverse Park Transform/1 -> "PWM Generator (Three-phase, Two-level)"/1(Vabc)
  Switch1/1 -> G/1
  Zero vector/1 -> Switch1/3
  PwmEnable/1 -> Unit Delay2/1
  "PWM Generator (Three-phase, Two-level)"/1(g) -> Switch1/1
  "PWM Generator (Three-phase, Two-level)"/2(ModWave) -> ModWave/1
  Mux/1 -> Scope/1, Inverse Park Transform/1
  vdqRef/1 -> Mux/1, Data Type Conversion Inherited/1
  theta/1 -> Inverse Park Transform/2

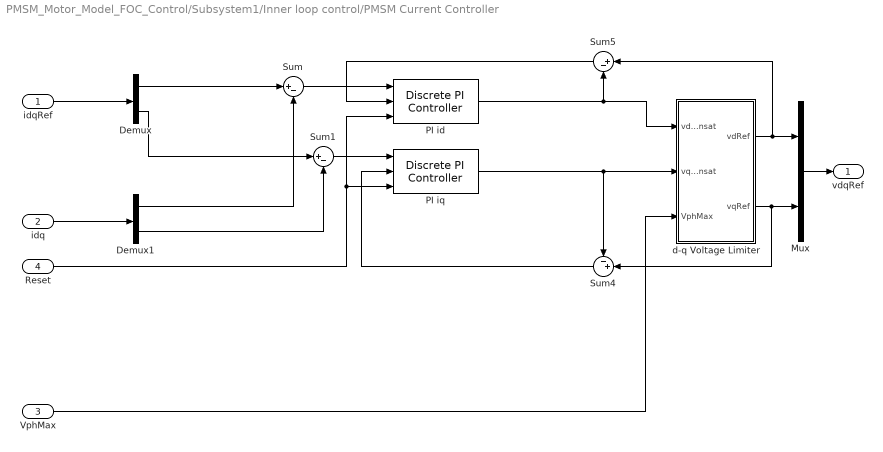
== system PMSM_Motor_Model_FOC_Control/Subsystem1/Inner loop control/PMSM Current Controller ==
  idqRef : Inport  SampleTime=Ts
  idq : Inport  Port=2  SampleTime=Ts
  VphMax : Inport  Port=3  SampleTime=Ts
  Reset : Inport  Port=4  SampleTime=Ts
  Demux : Demux  Outputs=2
  Demux1 : Demux  Outputs=2
  Mux : Mux  Inputs=2
  PI id : eeDiscretePi/Discrete PI Controller  Kp=Kp_id  Ki=Ki_id  Kaw=Kaw_id  x0=0  Ts=Ts
      settings: SourceProductBaseCode=PS
  PI iq : eeDiscretePi/Discrete PI Controller  Kp=Kp_iq  Ki=Ki_iq  Kaw=Kaw_iq  x0=0  Ts=Ts
      settings: SourceProductBaseCode=PS
  Sum : Sum  Inputs=|+-
  Sum1 : Sum  Inputs=|+-
  Sum4 : Sum  Inputs=-+|
  Sum5 : Sum  Inputs=|+-
  d-q Voltage Limiter : Subsystem  AncestorBlock=eeDqVoltageLimiter/d-q Voltage Limiter  LoadFcn=ee_sli_rtmsupport( 'loadfcn', gcbh );  mask(d-q Voltage Limiter){AxisPrio=Q-axis, Ts=Ts}
      mask prompts: AxisPrio "physmod:ee:library:comments:control:eeDqVoltageLimiter:AxisPrioritization_MP"; Ts "physmod:ee:library:comments:control:eeDqVoltageLimiter:SampleTime1ForInherited_MP"
      mask help: physmod:ee:library:comments:control:eeDqVoltageLimiter:dqVoltageLimiter_MD
      settings: CopyFcn=ee_sli_rtmsupport( 'copyfcn', gcbh );  DeleteFcn=ee_sli_rtmsupport( 'deletefcn', gcbh );  ModelCloseFcn=ee_sli_rtmsupport( 'modelclosefcn', gcbh );  PostSaveFcn=ee_sli_rtmsupport( 'postsavefcn', gcbh );  PreCopyFcn=ee_sli_rtmsupport( 'precopyfcn', gcbh );  OpenFcn=ee_sli_rtmsupport( 'openfcn', gcbh );  CloseFcn=ee_sli_rtmsupport( 'closefcn', gcbh );  PreDeleteFcn=ee_sli_rtmsupport( 'predeletefcn', gcbh );
      mask Help: web(nesl_help(gcbh))
      mask TypeOptions AxisPrio: physmod:ee:library:comments:control:eeDqVoltageLimiter:D0x2DAxis_PV | physmod:ee:library:comments:control:eeDqVoltageLimiter:Q0x2DAxis_PV | physmod:ee:library:comments:control:eeDqVoltageLimiter:D0x2DQEquivalence_PV
      mask DialogControl AxisPrio Prompt: Axis prioritization
      mask DialogControl Ts Prompt: Sample time (-1 for inherited)
  vdqRef : Outport  VectorParamsAs1DForOutWhenUnconnected=off
  wires:
  Mux/1 -> vdqRef/1
  Demux1/1 -> Sum/2
  d-q Voltage Limiter/1(vdRef) -> Sum5/1, Mux/1
  Sum/1 -> PI id/1
  Demux/1 -> Sum/1
  Sum4/1 -> PI iq/2
  PI iq/1 -> d-q Voltage Limiter/2(vqRefUnsat), Sum4/1
  PI id/1 -> d-q Voltage Limiter/1(vdRefUnsat), Sum5/2
  Sum1/1 -> PI iq/1
  Demux1/2 -> Sum1/2
  Sum5/1 -> PI id/2
  Demux/2 -> Sum1/1
  d-q Voltage Limiter/2(vqRef) -> Sum4/2, Mux/2
  idqRef/1 -> Demux/1
  idq/1 -> Demux1/1
  Reset/1 -> PI iq/3, PI id/3
  VphMax/1 -> d-q Voltage Limiter/3(VphMax)

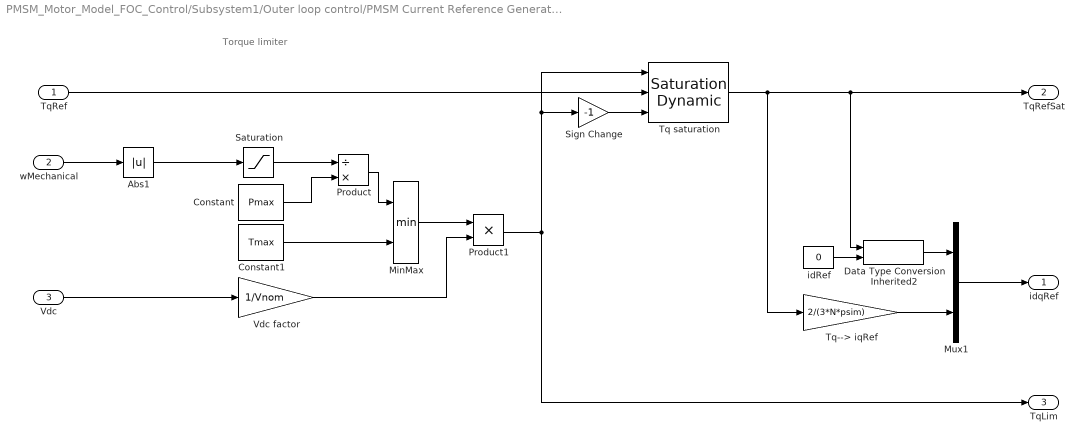
== system PMSM_Motor_Model_FOC_Control/Subsystem1/Outer loop control/PMSM Current Reference Generator ==
  note: Torque limiter
  TqRef : Inport  SampleTime=Ts
  wMechanical : Inport  Port=2  SampleTime=Ts
  Vdc : Inport  Port=3  SampleTime=Ts
  Abs1 : Abs
  Constant : Constant  Value=Pmax  SampleTime=Ts
  Constant1 : Constant  Value=Tmax  SampleTime=Ts
  Data Type Conversion Inherited2 : simulink/Signal Attributes/Data Type Conversion Inherited  ConvertRealWorld=Real World Value  DoSatur=off
      settings: SourceProductBaseCode=SL
  MinMax : MinMax  Inputs=2  OutDataTypeStr=Inherit: Same as first input
  Mux1 : Mux  Inputs=2
  Product : Product  Inputs=/*  OutDataTypeStr=Inherit: Same as first input
  Product1 : Product
  Saturation : Saturate  UpperLimit=inf  LowerLimit=Pmax/Tmax
  Sign Change : Gain  Gain=-1
  Tq saturation : simulink/Discontinuities/Saturation Dynamic  OutMin=[]  OutMax=[]  OutDataTypeStr=Inherit: Same as second input  OutDataType=fixdt(1, 16)  OutScaling=2^-10  DoSatur=off
  Tq--> iqRef : Gain  Gain=2/(3*N*psim)
  Vdc factor : Gain  Gain=1/Vnom
  idRef : Constant  Value=0  SampleTime=Ts
  idqRef : Outport  VectorParamsAs1DForOutWhenUnconnected=off
  TqRefSat : Outport  Port=2  VectorParamsAs1DForOutWhenUnconnected=off
  TqLim : Outport  Port=3  VectorParamsAs1DForOutWhenUnconnected=off
  wires:
  Vdc factor/1 -> Product1/2
  MinMax/1 -> Product1/1
  Sign Change/1 -> Tq saturation/3
  Product/1 -> MinMax/1
  Abs1/1 -> Saturation/1
  Constant1/1 -> MinMax/2
  Vdc/1 -> Vdc factor/1
  TqRef/1 -> Tq saturation/2
  Saturation/1 -> Product/1
  Constant/1 -> Product/2
  idRef/1 -> Data Type Conversion Inherited2/2
  Tq saturation/1 -> Tq--> iqRef/1, Data Type Conversion Inherited2/1, TqRefSat/1
  Product1/1 -> TqLim/1, Tq saturation/1, Sign Change/1
  Mux1/1 -> idqRef/1
  Data Type Conversion Inherited2/1 -> Mux1/1
  Tq--> iqRef/1 -> Mux1/2
  wMechanical/1 -> Abs1/1

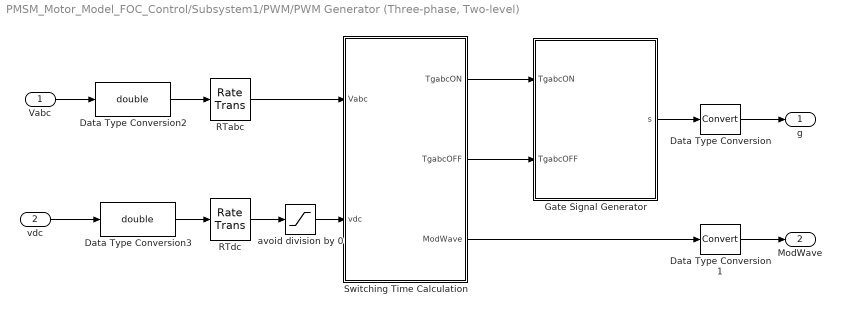
== system PMSM_Motor_Model_FOC_Control/Subsystem1/PWM/PWM Generator (Three-phase, Two-level) ==
  Vabc : Inport
  vdc : Inport  Port=2
  Data Type Conversion : DataTypeConversion
  Data Type Conversion1 : DataTypeConversion
  Data Type Conversion2 : DataTypeConversion  OutDataTypeStr=double
  Data Type Conversion3 : DataTypeConversion  OutDataTypeStr=double
  Gate Signal Generator : Subsystem
  RTabc : RateTransition  OutPortSampleTime=RateTransitionOnInput
  RTdc : RateTransition  OutPortSampleTime=RateTransitionOnInput
  Switching Time Calculation : MATLAB Function  TreatAsAtomicUnit=on
  avoid division by 0 : Saturate  UpperLimit=inf  LowerLimit=eps
  g : Outport  VectorParamsAs1DForOutWhenUnconnected=off
  ModWave : Outport  Port=2  VectorParamsAs1DForOutWhenUnconnected=off
  wires:
  Data Type Conversion3/1 -> RTdc/1
  Data Type Conversion2/1 -> RTabc/1
  vdc/1 -> Data Type Conversion3/1
  Vabc/1 -> Data Type Conversion2/1
  Switching Time Calculation/1(TgabcON) -> Gate Signal Generator/1(TgabcON)
  Switching Time Calculation/2(TgabcOFF) -> Gate Signal Generator/2(TgabcOFF)
  Gate Signal Generator/1(s) -> Data Type Conversion/1
  Data Type Conversion/1 -> g/1
  Switching Time Calculation/3(ModWave) -> Data Type Conversion1/1
  RTabc/1 -> Switching Time Calculation/1(Vabc)
  RTdc/1 -> avoid division by 0/1
  avoid division by 0/1 -> Switching Time Calculation/2(vdc)
  Data Type Conversion1/1 -> ModWave/1

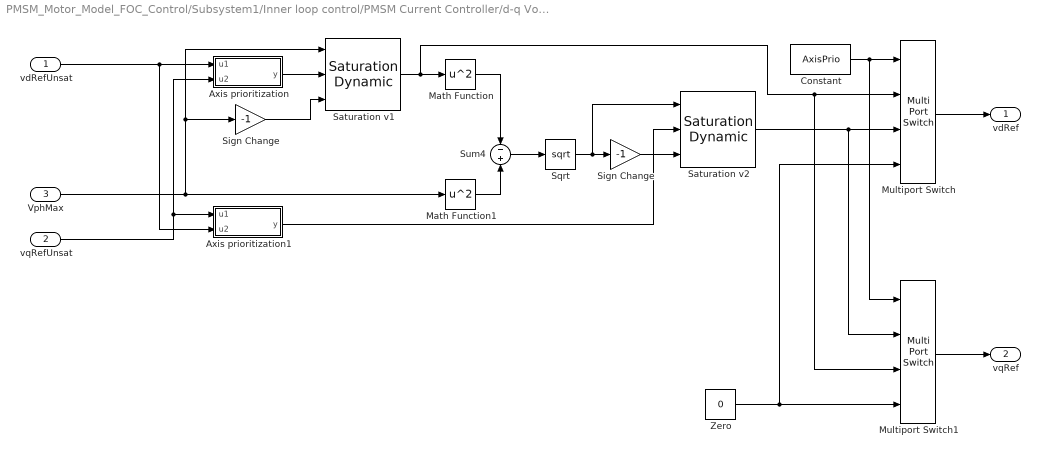
== system PMSM_Motor_Model_FOC_Control/Subsystem1/Inner loop control/PMSM Current Controller/d-q Voltage Limiter ==
  vdRefUnsat : Inport  SampleTime=Ts
  vqRefUnsat : Inport  Port=2  SampleTime=Ts
  VphMax : Inport  Port=3  SampleTime=Ts
  Axis prioritization : Subsystem
  Axis prioritization1 : Subsystem
  Constant : Constant  Value=AxisPrio  SampleTime=Ts
  Math Function : Math  Operator=square  SignedPower=on  SaturateOnIntegerOverflow=on
  Math Function1 : Math  Operator=square  SignedPower=on  SaturateOnIntegerOverflow=on
  Multiport Switch : MultiPortSwitch
  Multiport Switch1 : MultiPortSwitch
  Saturation v1 : simulink/Discontinuities/Saturation Dynamic  OutMin=[]  OutMax=[]  OutDataTypeStr=Inherit: Same as second input  OutDataType=fixdt(1, 16)  OutScaling=2^-10  DoSatur=off
  Saturation v2 : simulink/Discontinuities/Saturation Dynamic  OutMin=[]  OutMax=[]  OutDataTypeStr=Inherit: Same as second input  OutDataType=fixdt(1, 16)  OutScaling=2^-10  DoSatur=off
  Sign Change : Gain  Gain=-1
  "Sign Change " : Gain  Gain=-1
  Sqrt : Sqrt  SaturateOnIntegerOverflow=on
  Sum4 : Sum  Inputs=-+
  Zero : Constant  Value=0  OutDataTypeStr=Inherit: Inherit via back propagation
  vdRef : Outport  VectorParamsAs1DForOutWhenUnconnected=off
  vqRef : Outport  Port=2  VectorParamsAs1DForOutWhenUnconnected=off
  wires:
  Multiport Switch1/1 -> vqRef/1
  Multiport Switch/1 -> vdRef/1
  Saturation v2/1 -> Multiport Switch1/2, Multiport Switch/3
  Constant/1 -> Multiport Switch/1, Multiport Switch1/1
  vdRefUnsat/1 -> Axis prioritization1/2(u2), Axis prioritization/1(u1)
  VphMax/1 -> Sign Change/1, Saturation v1/1, Math Function1/1
  vqRefUnsat/1 -> Axis prioritization/2(u2), Axis prioritization1/1(u1)
  Axis prioritization/1(y) -> Saturation v1/2
  Axis prioritization1/1(y) -> Saturation v2/2
  Saturation v1/1 -> Math Function/1, Multiport Switch/2, Multiport Switch1/3
  Sign Change/1 -> Saturation v1/3
  Math Function1/1 -> Sum4/2
  Sum4/1 -> Sqrt/1
  Math Function/1 -> Sum4/1
  Sqrt/1 -> Saturation v2/1, "Sign Change "/1
  "Sign Change "/1 -> Saturation v2/3
  Zero/1 -> Multiport Switch1/4, Multiport Switch/4

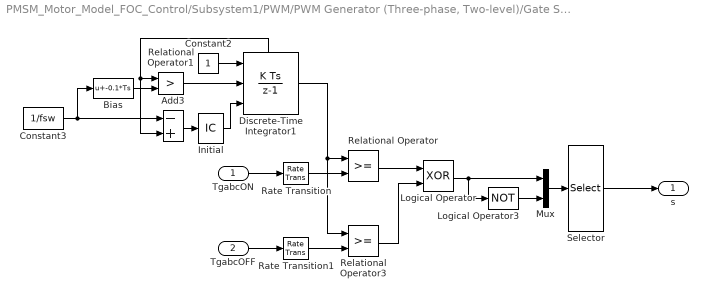
== system PMSM_Motor_Model_FOC_Control/Subsystem1/PWM/PWM Generator (Three-phase, Two-level)/Gate Signal Generator ==
  TgabcON : Inport
  TgabcOFF : Inport  Port=2
  Add3 : Sum  Inputs=-+
  Bias : Bias  Bias=-0.1*Ts
  Constant2 : Constant
  Constant3 : Constant  Value=1/fsw
  Discrete-Time Integrator1 : DiscreteIntegrator  ExternalReset=rising  InitialConditionSource=external  SampleTime=Ts  ShowStatePort=on  ICPrevOutput=DiscIntNeverNeededParam  ICPrevScaledInput=DiscIntNeverNeededParam
  Initial : InitialCondition  Value=GateGeneratorX0
  Logical Operator : Logic  Operator=XOR  AllPortsSameDT=off  OutDataTypeStr=boolean
  Logical Operator3 : Logic  Operator=NOT  AllPortsSameDT=off  OutDataTypeStr=boolean
  Mux : Mux  Inputs=2
  Rate Transition : RateTransition
  Rate Transition1 : RateTransition
  Relational Operator : RelationalOperator  OutDataTypeStr=boolean  RndMeth=Nearest
  Relational Operator1 : RelationalOperator  Operator=>  OutDataTypeStr=boolean  RndMeth=Nearest
  Relational Operator3 : RelationalOperator  OutDataTypeStr=boolean  RndMeth=Nearest
  Selector : Selector  InputPortWidth=6  IndexOptions=Index vector (dialog)  Indices=[1 4 2 5 3 6]  OutputSizes=1
  s : Outport  VectorParamsAs1DForOutWhenUnconnected=off
  wires:
  Relational Operator3/1 -> Logical Operator/2
  Relational Operator/1 -> Logical Operator/1
  Logical Operator/1 -> Logical Operator3/1, Mux/1
  Logical Operator3/1 -> Mux/2
  Mux/1 -> Selector/1
  Selector/1 -> s/1
  Discrete-Time Integrator1/1 -> Relational Operator3/1, Relational Operator/1
  Bias/1 -> Relational Operator1/2
  Relational Operator1/1 -> Discrete-Time Integrator1/2
  Add3/1 -> Initial/1
  Initial/1 -> Discrete-Time Integrator1/3
  Constant2/1 -> Discrete-Time Integrator1/1
  Discrete-Time Integrator1/State -> Add3/2, Relational Operator1/1
  Constant3/1 -> Bias/1, Add3/1
  TgabcON/1 -> Rate Transition/1
  TgabcOFF/1 -> Rate Transition1/1
  Rate Transition/1 -> Relational Operator/2
  Rate Transition1/1 -> Relational Operator3/2

== system PMSM_Motor_Model_FOC_Control/Subsystem1/Inner loop control/PMSM Current Controller/d-q Voltage Limiter/Axis prioritization ==
  u1 : Inport
  u2 : Inport  Port=2
  Compare To Constant : simulink/Logic and Bit Operations/Compare To Constant  relop===  const=1  OutDataTypeStr=boolean
  Constant : Constant  Value=AxisPrio  SampleTime=Ts
  Switch : Switch  Criteria=u2 ~= 0  Threshold=1
  y : Outport  VectorParamsAs1DForOutWhenUnconnected=off
  wires:
  Compare To Constant/1 -> Switch/2
  Constant/1 -> Compare To Constant/1
  Switch/1 -> y/1
  u2/1 -> Switch/3
  u1/1 -> Switch/1

== system PMSM_Motor_Model_FOC_Control/Subsystem1/Inner loop control/PMSM Current Controller/d-q Voltage Limiter/Axis prioritization1 ==
  u1 : Inport
  u2 : Inport  Port=2
  Compare To Constant : simulink/Logic and Bit Operations/Compare To Constant  relop===  const=1  OutDataTypeStr=boolean
  Constant : Constant  Value=AxisPrio  SampleTime=Ts
  Switch : Switch  Criteria=u2 ~= 0  Threshold=1
  y : Outport  VectorParamsAs1DForOutWhenUnconnected=off
  wires:
  Constant/1 -> Compare To Constant/1
  Compare To Constant/1 -> Switch/2
  Switch/1 -> y/1
  u2/1 -> Switch/3
  u1/1 -> Switch/1

== matlab function PMSM_Motor_Model_FOC_Control/Subsystem1/PWM/PWM Generator (Three-phase, Two-level)/Switching Time Calculation ==
  settings: sampleTime=1
  data: Vabc input; TgabcON output; vdc input; TgabcOFF output; ModWave output; fsw parameter; PWM parameter
function [TgabcON,TgabcOFF,ModWave]  = switchingTime(Vabc,vdc,fsw,PWM)

[TgabcON,TgabcOFF,ModWave] = ee.control.pwmSwitchingTimeTwoLevel(Vabc,vdc,fsw,PWM);
